simulink model "lab1_2"  (R2020b)
settings: Solver=VariableStepAuto  StartTime=0.0  StopTime=100.0  RelTol=10e-10  AbsTol=10e-10
values from neighbouring files (symbols this model uses):
  den1 = cell2mat(den1)    [lab1.m]
  num1 = cell2mat(num1)    [lab1.m]
settings Model: Creator=jiayizhou  LastModifiedBy=jiayizhou

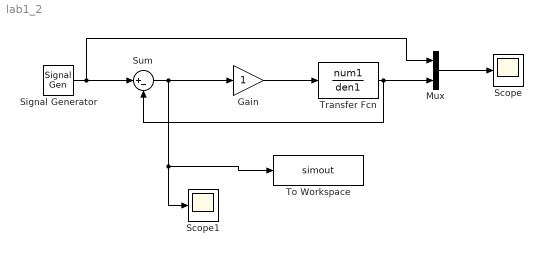
== system lab1_2 ==
  Gain : Gain
  Mux : Mux  Inputs=2
  Scope : Scope
  Scope1 : Scope
  Signal Generator : SignalGenerator  WaveForm=square  Frequency=0.02
  Sum : Sum  Inputs=|+-
  To Workspace : ToWorkspace  VariableName=simout  SaveFormat=Timeseries  SampleTime=-1
  Transfer Fcn : TransferFcn  Numerator=num1  Denominator=den1
  wires:
  Sum/1 -> To Workspace/1, Scope1/1, Gain/1
  Gain/1 -> Transfer Fcn/1
  Transfer Fcn/1 -> Sum/2, Mux/2
  Signal Generator/1 -> Mux/1, Sum/1
  Mux/1 -> Scope/1
